simulink model "ilcPathOpt_th"  (R2022a)
settings: Solver=FixedStepAuto  StartTime=0.0  StopTime=duration_s  FixedStep=0.001  RelTol=1e-3
values from neighbouring files (symbols this model uses):
  coeffs = [1 0 -1 0 -1]    [ilcPathOpt_ts.m]
libraries: ilcPathOpt_cl x1
settings Model: Creator=mcobb  LastModifiedBy=lhill8
settings SolverCC: AlgebraicLoopSolver=TrustRegion
settings DebuggingCC: UnconnectedInputMsg=warning  UnconnectedOutputMsg=warning  UnconnectedLineMsg=warning  SFMachineParentedDataDiag=warning  ArithmeticOperatorsInVariantConditions=warning
settings SFSimCC: CustomCodeUndefinedFunction=UseInterfaceOnly

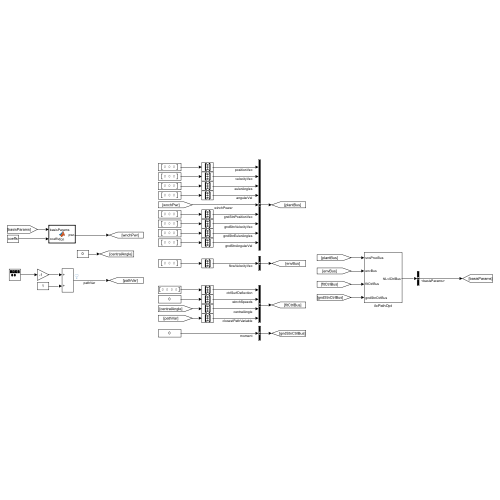
[thumbnail: Simulink's stored preview of the top-level diagram]
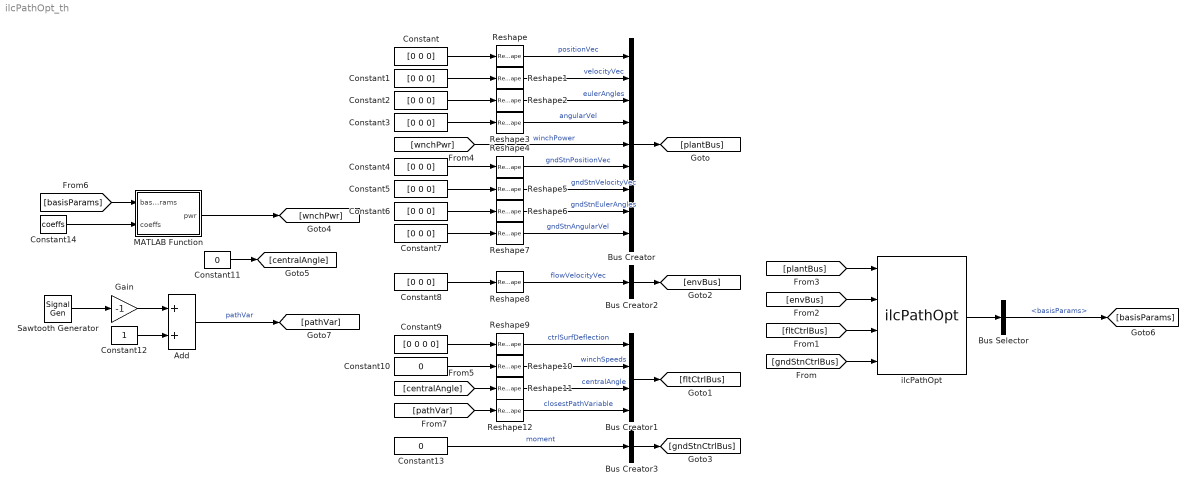
== system ilcPathOpt_th ==
  Add : Sum
  Bus Creator : BusCreator  Inputs=9  OutDataTypeStr=Bus: plantBus
  Bus Creator1 : BusCreator  Inputs=4  OutDataTypeStr=Bus: fltCtrlBus
  Bus Creator2 : BusCreator  Inputs=1  OutDataTypeStr=Bus: envBus
  Bus Creator3 : BusCreator  Inputs=1  OutDataTypeStr=Bus: gndStnCtrlBus
  Bus Selector : BusSelector  OutputSignals=basisParams
  Constant{,1..8} (9 alike) : Constant  Value=[0 0 0]
  Constant10 : Constant  Value=0
  Constant11 : Constant  Value=0
  Constant12 : Constant
  Constant13 : Constant  Value=0
  Constant14 : Constant  Value=coeffs
  Constant9 : Constant  Value=[0 0 0 0]
  Gain : Gain  Gain=-1
  MATLAB Function : MATLAB Function  TreatAsAtomicUnit=on
  Reshape{,1..12} (13 alike) : Reshape  OutputDimensionality=Column vector (2-D)
  Sawtooth Generator : SignalGenerator  WaveForm=sawtooth
  ilcPathOpt : ilcPathOpt_cl/ilcPathOpt  ctrl=hiLvlCtrl
  wires:
  Bus Creator/1 -> [plantBus]
  Bus Creator1/1 -> [fltCtrlBus]
  Bus Creator2/1 -> [envBus]
  Bus Creator3/1 -> [gndStnCtrlBus]
  [gndStnCtrlBus] -> ilcPathOpt/4
  [fltCtrlBus] -> ilcPathOpt/3
  [envBus] -> ilcPathOpt/2
  [plantBus] -> ilcPathOpt/1
  ilcPathOpt/1 -> Bus Selector/1
  Constant/1 -> Reshape/1
  Reshape/1 -> Bus Creator/1  "positionVec"
  Constant1/1 -> Reshape1/1
  Reshape1/1 -> Bus Creator/2  "velocityVec"
  Constant2/1 -> Reshape2/1
  Reshape2/1 -> Bus Creator/3  "eulerAngles"
  Constant3/1 -> Reshape3/1
  Reshape3/1 -> Bus Creator/4  "angularVel"
  Constant4/1 -> Reshape4/1
  Reshape4/1 -> Bus Creator/6  "gndStnPositionVec"
  Constant5/1 -> Reshape5/1
  Reshape5/1 -> Bus Creator/7  "gndStnVelocityVec"
  Constant6/1 -> Reshape6/1
  Reshape6/1 -> Bus Creator/8  "gndStnEulerAngles"
  Constant7/1 -> Reshape7/1
  Reshape7/1 -> Bus Creator/9  "gndStnAngularVel"
  [wnchPwr] -> Bus Creator/5  "winchPower"
  Reshape8/1 -> Bus Creator2/1  "flowVelocityVec"
  Constant8/1 -> Reshape8/1
  Constant9/1 -> Reshape9/1
  Reshape9/1 -> Bus Creator1/1  "ctrlSurfDeflection"
  Reshape10/1 -> Bus Creator1/2  "winchSpeeds"
  Constant10/1 -> Reshape10/1
  Reshape11/1 -> Bus Creator1/3  "centralAngle"
  [centralAngle] -> Reshape11/1
  Reshape12/1 -> Bus Creator1/4  "closestPathVariable"
  [pathVar] -> Reshape12/1
  Constant13/1 -> Bus Creator3/1  "moment"
  Constant11/1 -> [centralAngle]
  Bus Selector/1 -> [basisParams]  "<basisParams>"
  [basisParams] -> MATLAB Function/1(basisParams)
  Constant14/1 -> MATLAB Function/2(coeffs)
  MATLAB Function/1(pwr) -> [wnchPwr]
  Sawtooth Generator/1 -> Gain/1
  Constant12/1 -> Add/2
  Add/1 -> [pathVar]  "pathVar"
  Gain/1 -> Add/1

== matlab function ilcPathOpt_th/MATLAB Function ==
  data: basisParams input; pwr output; coeffs input
function pwr = fcn(basisParams,coeffs)

pwr = coeffs(1)+...
    coeffs(2)*basisParams(1)+...
    coeffs(3)*basisParams(1).^2+...
    coeffs(4)*basisParams(2)+...
    coeffs(5)*basisParams(2).^2;
